simulink model "PID_controller"  (R2020b)
settings: Solver=VariableStepAuto  StartTime=0.0  StopTime=10.0  RelTol=1e-3
settings Model: Creator=adima  LastModifiedBy=adima

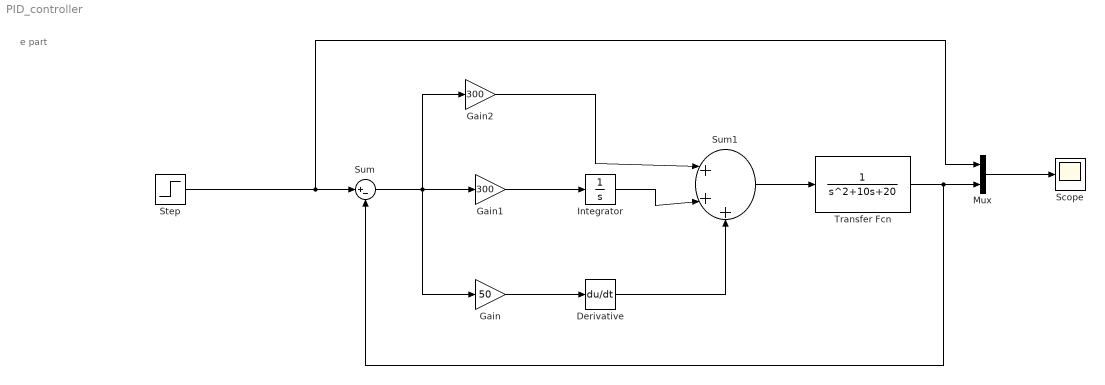
== system PID_controller ==
  note: e part
  Derivative : Derivative
  Gain : Gain  Gain=50
  Gain1 : Gain  Gain=300
  Gain2 : Gain  Gain=300
  Integrator : Integrator
  Mux : Mux  Inputs=2
  Scope : Scope
  Step : Step  SampleTime=0
  Sum : Sum  Inputs=|+-
  Sum1 : Sum  Inputs=|+++
  Transfer Fcn : TransferFcn  Denominator=[1 10 20]
  wires:
  Step/1 -> Mux/1, Sum/1
  Sum/1 -> Gain1/1, Gain/1, Gain2/1
  Gain/1 -> Derivative/1
  Derivative/1 -> Sum1/3
  Gain2/1 -> Sum1/1
  Sum1/1 -> Transfer Fcn/1
  Mux/1 -> Scope/1
  Transfer Fcn/1 -> Sum/2, Mux/2
  Gain1/1 -> Integrator/1
  Integrator/1 -> Sum1/2
